simulink library "EmE_MBD_Blockset"  (R2018a)
settings: Solver=ode1  StartTime=0.0  StopTime=Inf  FixedStep=0.001  RelTol=1e-3  EnableMultiTasking=on
PostLoadFcn:
  | , if any(exist('dsrtsu_mdlpostloadfcn', 'file') == [2, 3, 6]), try dsrtsu_mdlpostloadfcn('Execute', bdroot); catch fprintf('Error in PostLoadFcn (dsrtsu_mdlpostloadfcn) for model "%s":\n %s\n', bdroot, lasterr); end, end,
undefined symbols (not defined in the file or in its folder): ENUM_TSC1_CONTROL_PURPOSE_T, gcbh, GLB_SWITCH_T
libraries: simulink x237, $bdroot x115, simulink_need_slupdate x26, MotoHawk_lib x13, simulink_extras x3
(part 11 of 11)

== system EmE_MBD_Blockset/User-Defined Functions/Snoop/CCP_ETC_SS2/CCP_Parameter_Decode/Decode_Signal7/Signal Decode/FLOAT32 ==
  note: (-1)^s × c × b^q
  note: S        Q         C
      | 31    30-23    22-0
  Raw32 : Inport
  Add8 : Sum
  Add9 : Sum  Inputs=-+
  Bitwise Operator : simulink/Logic and Bit Operations/Bitwise Operator  logicop=AND  UseBitMask=on  BitMask=bin2dec('10000000000000000000000000000000')  BitMaskRealWorld=Stored Integer
  Bitwise Operator1 : simulink/Logic and Bit Operations/Bitwise Operator  logicop=AND  UseBitMask=on  BitMask=bin2dec('01111111100000000000000000000000')  BitMaskRealWorld=Stored Integer
  Bitwise Operator2 : simulink/Logic and Bit Operations/Bitwise Operator  logicop=AND  UseBitMask=on  BitMask=bin2dec('00000000011111111111111111111111')  BitMaskRealWorld=Stored Integer
  Constant : Constant  Value=10
  Constant5 : Constant  OutDataTypeStr=double
  Constant6 : Constant  Value=2  OutDataTypeStr=double
  Constant7 : Constant  Value=127  OutDataTypeStr=double
  Data Type Conversion{1..8} (8 alike) : DataTypeConversion  OutDataTypeStr=double
  Math Function1 : Math  Operator=pow  SaturateOnIntegerOverflow=on
  Product1 : Product  RndMeth=Zero
  Shift Arithmetic6 : ArithShift
  Shift Arithmetic7 : ArithShift
  Shift Arithmetic8 : ArithShift
  Terminator3 : Terminator
  sign1 : Terminator
  Raw : Outport
  wires:
  Data Type Conversion8/1 -> Product1/1
  Data Type Conversion7/1 -> Product1/2
  Data Type Conversion6/1 -> Add8/1
  Data Type Conversion5/1 -> Add9/1
  Data Type Conversion3/1 -> Shift Arithmetic8/1
  Data Type Conversion1/1 -> Raw/1
  Product1/1 -> Data Type Conversion1/1
  Add8/1 -> Data Type Conversion7/1
  Constant7/1 -> Data Type Conversion5/1
  Data Type Conversion4/1 -> Add9/2
  Math Function1/1 -> Data Type Conversion8/1
  Constant6/1 -> Math Function1/1
  Add9/1 -> Math Function1/2
  Shift Arithmetic7/1 -> Data Type Conversion4/1
  Data Type Conversion2/1 -> Add8/2
  Constant5/1 -> Data Type Conversion6/1
  Shift Arithmetic8/1 -> Data Type Conversion2/1
  Shift Arithmetic6/1 -> sign1/1
  Bitwise Operator/1 -> Shift Arithmetic6/1  "s"
  Bitwise Operator1/1 -> Shift Arithmetic7/1  "q"
  Bitwise Operator2/1 -> Data Type Conversion3/1  "c"
  Raw32/1 -> Bitwise Operator/1, Bitwise Operator1/1, Bitwise Operator2/1
  Constant/1 -> Terminator3/1  "b"

== system EmE_MBD_Blockset/User-Defined Functions/Snoop/CCP_ETC_SS2/CCP_Parameter_Decode/Decode_Signal7/Signal Decode/Integer_Data ==
  Type : Inport
  Raw32 : Inport  Port=2
  Bitwise Operator : simulink/Logic and Bit Operations/Bitwise Operator  logicop=AND  UseBitMask=on  BitMask=bin2dec('1000')  BitMaskRealWorld=Stored Integer
  Bitwise Operator1 : simulink/Logic and Bit Operations/Bitwise Operator  logicop=AND  UseBitMask=on  BitMask=hex2dec('8000')  BitMaskRealWorld=Stored Integer
  Bitwise Operator2 : simulink/Logic and Bit Operations/Bitwise Operator  logicop=AND  UseBitMask=on  BitMask=bin2dec('0100')  BitMaskRealWorld=Stored Integer
  Bitwise Operator3 : simulink/Logic and Bit Operations/Bitwise Operator  logicop=AND  UseBitMask=on  BitMask=bin2dec('0010')  BitMaskRealWorld=Stored Integer
  Bitwise Operator5 : simulink/Logic and Bit Operations/Bitwise Operator  logicop=AND  UseBitMask=on  BitMask=hex2dec('80')  BitMaskRealWorld=Stored Integer
  Bitwise Operator6 : simulink/Logic and Bit Operations/Bitwise Operator  logicop=AND  UseBitMask=on  BitMask=hex2dec('80000000')  BitMaskRealWorld=Stored Integer
  Bitwise Operator7 : simulink/Logic and Bit Operations/Bitwise Operator  logicop=AND  UseBitMask=on  BitMask=bin2dec('0111111111111111')  BitMaskRealWorld=Stored Integer
  Bitwise Operator8 : simulink/Logic and Bit Operations/Bitwise Operator  logicop=AND  UseBitMask=on  BitMask=hex2dec('7F')  BitMaskRealWorld=Stored Integer
  Bitwise Operator9 : simulink/Logic and Bit Operations/Bitwise Operator  logicop=AND  UseBitMask=on  BitMask=hex2dec('7FFFFFF')  BitMaskRealWorld=Stored Integer
  Constant1 : Constant  Value=0  OutDataTypeStr=boolean
  Constant3 : Constant  OutDataTypeStr=boolean
  Data Type Conversion{5,9..11} (4 alike) : DataTypeConversion  OutDataTypeStr=double
  Gain : Gain  Gain=-1
  Logical Operator{,2..4} (4 alike) : Logic  AllPortsSameDT=off  OutDataTypeStr=boolean
  Logical Operator1 : Logic  Operator=NOR  AllPortsSameDT=off  OutDataTypeStr=boolean
  Logical Operator5 : Logic  Operator=OR  Inputs=3  AllPortsSameDT=off  OutDataTypeStr=boolean
  Switch{1..5} (5 alike) : Switch  Criteria=u2 ~= 0
  Raw : Outport
  wires:
  Type/1 -> Bitwise Operator/1, Bitwise Operator3/1, Bitwise Operator2/1
  Bitwise Operator/1 -> Switch1/2  "F_signed"
  Constant3/1 -> Switch1/1
  Constant1/1 -> Switch1/3
  Switch1/1 -> [f_signed]  "Sign"
  [f_signed] -> Switch4/2
  Switch5/1 -> Raw/1
  Bitwise Operator2/1 -> [F_4Byte], Logical Operator1/1  "F_4Byte"
  Bitwise Operator3/1 -> [F_2Byte], Logical Operator1/2  "F_2Byte"
  Logical Operator1/1 -> [F_1Byte]
  Bitwise Operator5/1 -> Logical Operator/2
  Bitwise Operator1/1 -> Logical Operator3/2
  Bitwise Operator6/1 -> Logical Operator4/2
  Raw32/1 -> Bitwise Operator5/1, Bitwise Operator6/1, Bitwise Operator1/1, Bitwise Operator8/1, Bitwise Operator7/1, Bitwise Operator9/1, Data Type Conversion10/1
  Bitwise Operator7/1 -> Data Type Conversion9/1
  Data Type Conversion9/1 -> Switch2/1
  [F_2Byte] -> Switch2/2
  Bitwise Operator8/1 -> Data Type Conversion5/1
  Data Type Conversion5/1 -> Switch2/3
  [F_1Byte] -> Logical Operator/1
  [F_2Byte] -> Logical Operator3/1
  [F_4Byte] -> Logical Operator4/1
  Logical Operator/1 -> Logical Operator5/1
  Logical Operator3/1 -> Logical Operator5/2
  Logical Operator4/1 -> Logical Operator5/3
  Logical Operator5/1 -> [flip_sign]  "flip_sign"
  Switch2/1 -> Switch3/3
  [F_4Byte] -> Switch3/2
  Data Type Conversion10/1 -> Switch4/3
  Bitwise Operator9/1 -> Data Type Conversion11/1
  Data Type Conversion11/1 -> Switch3/1
  Switch3/1 -> Switch4/1
  Gain/1 -> Switch5/1
  Switch4/1 -> Switch5/3, Gain/1
  Logical Operator2/1 -> Switch5/2
  [flip_sign] -> Logical Operator2/2
  [f_signed] -> Logical Operator2/1

== system EmE_MBD_Blockset/User-Defined Functions/Snoop/CCP_ETC_SS2/CCP_Parameter_Decode/Decode_Signal7/Signal Decode/Unit_Convert ==
  Raw : Inport
  Conversion : Inport  Port=2
  Add : Sum
  Divide : Product  Inputs=*/
  Product : Product  RndMeth=Zero
  Selector1 : Selector  InputPortWidth=3  IndexOptions=Index vector (dialog)  Indices=3  OutputSizes=1
  Selector2 : Selector  InputPortWidth=3  IndexOptions=Index vector (dialog)  Indices=1  OutputSizes=1
  Selector4 : Selector  InputPortWidth=3  IndexOptions=Index vector (dialog)  Indices=2  OutputSizes=1
  Scaled : Outport
  wires:
  Add/1 -> Scaled/1
  Divide/1 -> Add/1
  Product/1 -> Divide/1
  Selector2/1 -> Product/2
  Selector4/1 -> Divide/2
  Selector1/1 -> Add/2
  Conversion/1 -> Selector2/1, Selector4/1, Selector1/1
  Raw/1 -> Product/1

== system EmE_MBD_Blockset/User-Defined Functions/Snoop/CCP_ETC_SS2/CCP_Parameter_Decode/Decode_Signal8/Isolate Data/1Byte ==
  U : Inport
  Idx : Inport  Port=2
  1Byte : Selector  IndexMode=Zero-based  InputPortWidth=7  IndexOptions=Starting index (port)  Indices=1  OutputSizes=1
  Data Type Conversion : DataTypeConversion  OutDataTypeStr=uint32
  Y : Outport
  wires:
  Data Type Conversion/1 -> Y/1
  Idx/1 -> 1Byte/2
  1Byte/1 -> Data Type Conversion/1
  U/1 -> 1Byte/1

== system EmE_MBD_Blockset/User-Defined Functions/Snoop/CCP_ETC_SS2/CCP_Parameter_Decode/Decode_Signal8/Isolate Data/2Bytes ==
  U : Inport
  Idx1 : Inport  Port=2
  2Byte : Selector  IndexMode=Zero-based  InputPortWidth=7  IndexOptions=Starting index (port)  Indices=1  OutputSizes=2
  Add : Sum
  Constant : Constant  Value=5  OutDataTypeStr=uint8
  Data Type Conversion : DataTypeConversion  OutDataTypeStr=uint32
  Data Type Conversion1 : DataTypeConversion  OutDataTypeStr=uint32
  Demux : Demux  Outputs=2
  Relational Operator : RelationalOperator  Operator=<  OutDataTypeStr=boolean  RndMeth=Nearest
  Shift Arithmetic : ArithShift
  Switch1 : Switch  Criteria=u2 ~= 0
  Y : Outport
  wires:
  Switch1/1 -> 2Byte/2
  Idx1/1 -> Switch1/3, Relational Operator/2
  Relational Operator/1 -> Switch1/2
  2Byte/1 -> Data Type Conversion1/1
  Data Type Conversion1/1 -> Demux/1
  Add/1 -> Data Type Conversion/1
  Shift Arithmetic/1 -> Add/1
  Demux/1 -> Shift Arithmetic/1
  Demux/2 -> Add/2
  U/1 -> 2Byte/1
  Data Type Conversion/1 -> Y/1
  Constant/1 -> Switch1/1, Relational Operator/1

== system EmE_MBD_Blockset/User-Defined Functions/Snoop/CCP_ETC_SS2/CCP_Parameter_Decode/Decode_Signal8/Isolate Data/4Bytes ==
  U : Inport
  Idx : Inport  Port=2
  4Byte : Selector  IndexMode=Zero-based  InputPortWidth=7  IndexOptions=Starting index (port)  Indices=1  OutputSizes=4
  Add : Sum  Inputs=++++
  Constant1 : Constant  Value=3  OutDataTypeStr=uint8
  Data Type Conversion1 : DataTypeConversion  OutDataTypeStr=uint32
  Data Type Conversion2 : DataTypeConversion  OutDataTypeStr=uint32
  Demux : Demux
  Relational Operator1 : RelationalOperator  Operator=<  OutDataTypeStr=boolean  RndMeth=Nearest
  Shift Arithmetic : ArithShift
  Shift Arithmetic1 : ArithShift
  Shift Arithmetic2 : ArithShift
  Switch2 : Switch  Criteria=u2 ~= 0
  Y : Outport
  wires:
  Switch2/1 -> 4Byte/2
  Data Type Conversion2/1 -> Demux/1
  Shift Arithmetic2/1 -> Add/3
  Demux/3 -> Shift Arithmetic2/1
  Demux/4 -> Add/4
  Shift Arithmetic1/1 -> Add/2
  Add/1 -> Data Type Conversion1/1
  Shift Arithmetic/1 -> Add/1
  Demux/1 -> Shift Arithmetic/1
  Demux/2 -> Shift Arithmetic1/1
  Data Type Conversion1/1 -> Y/1
  4Byte/1 -> Data Type Conversion2/1
  U/1 -> 4Byte/1
  Idx/1 -> Switch2/3, Relational Operator1/2
  Relational Operator1/1 -> Switch2/2
  Constant1/1 -> Switch2/1, Relational Operator1/1

== system EmE_MBD_Blockset/User-Defined Functions/Snoop/CCP_ETC_SS2/CCP_Parameter_Decode/Decode_Signal8/Isolate Data/Size ==
  Type : Inport
  Bitwise Operator : simulink/Logic and Bit Operations/Bitwise Operator  logicop=AND  UseBitMask=on  BitMask=bin2dec('00000001')  BitMaskRealWorld=Stored Integer
  Bitwise Operator1 : simulink/Logic and Bit Operations/Bitwise Operator  logicop=AND  UseBitMask=on  BitMask=bin2dec('00000010')  BitMaskRealWorld=Stored Integer
  Bitwise Operator2 : simulink/Logic and Bit Operations/Bitwise Operator  logicop=AND  UseBitMask=on  BitMask=bin2dec('00000100')  BitMaskRealWorld=Stored Integer
  Constant2 : Constant  Value=2
  Constant3 : Constant
  Constant4 : Constant  Value=4
  Logical Operator : Logic  Operator=OR  AllPortsSameDT=off  OutDataTypeStr=boolean
  Logical Operator1 : Logic  Operator=NOT  AllPortsSameDT=off  OutDataTypeStr=boolean
  Switch1 : Switch  Criteria=u2 ~= 0
  Switch2 : Switch  Criteria=u2 ~= 0
  Byte_Count : Outport
  wires:
  Constant4/1 -> Switch2/1
  Switch2/1 -> Byte_Count/1
  Constant3/1 -> Switch1/3
  Constant2/1 -> Switch1/1
  Bitwise Operator1/1 -> Switch1/2
  Logical Operator1/1 -> Logical Operator/1
  Bitwise Operator2/1 -> Logical Operator/2
  Switch1/1 -> Switch2/3
  Bitwise Operator/1 -> Logical Operator1/1
  Type/1 -> Bitwise Operator/1, Bitwise Operator1/1, Bitwise Operator2/1
  Logical Operator/1 -> Switch2/2

== system EmE_MBD_Blockset/User-Defined Functions/Snoop/CCP_ETC_SS2/CCP_Parameter_Decode/Decode_Signal8/Signal Decode/FLOAT32 ==
  note: S        Q         C
      | 31    30-23    22-0
  note: (-1)^s × c × b^q
  Raw32 : Inport
  Add8 : Sum
  Add9 : Sum  Inputs=-+
  Bitwise Operator : simulink/Logic and Bit Operations/Bitwise Operator  logicop=AND  UseBitMask=on  BitMask=bin2dec('10000000000000000000000000000000')  BitMaskRealWorld=Stored Integer
  Bitwise Operator1 : simulink/Logic and Bit Operations/Bitwise Operator  logicop=AND  UseBitMask=on  BitMask=bin2dec('01111111100000000000000000000000')  BitMaskRealWorld=Stored Integer
  Bitwise Operator2 : simulink/Logic and Bit Operations/Bitwise Operator  logicop=AND  UseBitMask=on  BitMask=bin2dec('00000000011111111111111111111111')  BitMaskRealWorld=Stored Integer
  Constant : Constant  Value=10
  Constant5 : Constant  OutDataTypeStr=double
  Constant6 : Constant  Value=2  OutDataTypeStr=double
  Constant7 : Constant  Value=127  OutDataTypeStr=double
  Data Type Conversion{1..8} (8 alike) : DataTypeConversion  OutDataTypeStr=double
  Math Function1 : Math  Operator=pow  SaturateOnIntegerOverflow=on
  Product1 : Product  RndMeth=Zero
  Shift Arithmetic6 : ArithShift
  Shift Arithmetic7 : ArithShift
  Shift Arithmetic8 : ArithShift
  Terminator3 : Terminator
  sign1 : Terminator
  Raw : Outport
  wires:
  Constant/1 -> Terminator3/1  "b"
  Raw32/1 -> Bitwise Operator2/1, Bitwise Operator1/1, Bitwise Operator/1
  Bitwise Operator2/1 -> Data Type Conversion3/1  "c"
  Bitwise Operator1/1 -> Shift Arithmetic7/1  "q"
  Bitwise Operator/1 -> Shift Arithmetic6/1  "s"
  Shift Arithmetic6/1 -> sign1/1
  Shift Arithmetic8/1 -> Data Type Conversion2/1
  Constant5/1 -> Data Type Conversion6/1
  Data Type Conversion2/1 -> Add8/2
  Shift Arithmetic7/1 -> Data Type Conversion4/1
  Add9/1 -> Math Function1/2
  Constant6/1 -> Math Function1/1
  Math Function1/1 -> Data Type Conversion8/1
  Data Type Conversion4/1 -> Add9/2
  Constant7/1 -> Data Type Conversion5/1
  Add8/1 -> Data Type Conversion7/1
  Product1/1 -> Data Type Conversion1/1
  Data Type Conversion1/1 -> Raw/1
  Data Type Conversion3/1 -> Shift Arithmetic8/1
  Data Type Conversion5/1 -> Add9/1
  Data Type Conversion6/1 -> Add8/1
  Data Type Conversion7/1 -> Product1/2
  Data Type Conversion8/1 -> Product1/1

== system EmE_MBD_Blockset/User-Defined Functions/Snoop/CCP_ETC_SS2/CCP_Parameter_Decode/Decode_Signal8/Signal Decode/Integer_Data ==
  Type : Inport
  Raw32 : Inport  Port=2
  Bitwise Operator : simulink/Logic and Bit Operations/Bitwise Operator  logicop=AND  UseBitMask=on  BitMask=bin2dec('1000')  BitMaskRealWorld=Stored Integer
  Bitwise Operator1 : simulink/Logic and Bit Operations/Bitwise Operator  logicop=AND  UseBitMask=on  BitMask=hex2dec('8000')  BitMaskRealWorld=Stored Integer
  Bitwise Operator2 : simulink/Logic and Bit Operations/Bitwise Operator  logicop=AND  UseBitMask=on  BitMask=bin2dec('0100')  BitMaskRealWorld=Stored Integer
  Bitwise Operator3 : simulink/Logic and Bit Operations/Bitwise Operator  logicop=AND  UseBitMask=on  BitMask=bin2dec('0010')  BitMaskRealWorld=Stored Integer
  Bitwise Operator5 : simulink/Logic and Bit Operations/Bitwise Operator  logicop=AND  UseBitMask=on  BitMask=hex2dec('80')  BitMaskRealWorld=Stored Integer
  Bitwise Operator6 : simulink/Logic and Bit Operations/Bitwise Operator  logicop=AND  UseBitMask=on  BitMask=hex2dec('80000000')  BitMaskRealWorld=Stored Integer
  Bitwise Operator7 : simulink/Logic and Bit Operations/Bitwise Operator  logicop=AND  UseBitMask=on  BitMask=bin2dec('0111111111111111')  BitMaskRealWorld=Stored Integer
  Bitwise Operator8 : simulink/Logic and Bit Operations/Bitwise Operator  logicop=AND  UseBitMask=on  BitMask=hex2dec('7F')  BitMaskRealWorld=Stored Integer
  Bitwise Operator9 : simulink/Logic and Bit Operations/Bitwise Operator  logicop=AND  UseBitMask=on  BitMask=hex2dec('7FFFFFF')  BitMaskRealWorld=Stored Integer
  Constant1 : Constant  Value=0  OutDataTypeStr=boolean
  Constant3 : Constant  OutDataTypeStr=boolean
  Data Type Conversion{5,9..11} (4 alike) : DataTypeConversion  OutDataTypeStr=double
  Gain : Gain  Gain=-1
  Logical Operator{,2..4} (4 alike) : Logic  AllPortsSameDT=off  OutDataTypeStr=boolean
  Logical Operator1 : Logic  Operator=NOR  AllPortsSameDT=off  OutDataTypeStr=boolean
  Logical Operator5 : Logic  Operator=OR  Inputs=3  AllPortsSameDT=off  OutDataTypeStr=boolean
  Switch{1..5} (5 alike) : Switch  Criteria=u2 ~= 0
  Raw : Outport
  wires:
  [f_signed] -> Logical Operator2/1
  [flip_sign] -> Logical Operator2/2
  Logical Operator2/1 -> Switch5/2
  Switch4/1 -> Gain/1, Switch5/3
  Gain/1 -> Switch5/1
  Switch3/1 -> Switch4/1
  Data Type Conversion11/1 -> Switch3/1
  Bitwise Operator9/1 -> Data Type Conversion11/1
  Data Type Conversion10/1 -> Switch4/3
  [F_4Byte] -> Switch3/2
  Switch2/1 -> Switch3/3
  Logical Operator5/1 -> [flip_sign]  "flip_sign"
  Logical Operator4/1 -> Logical Operator5/3
  Logical Operator3/1 -> Logical Operator5/2
  Logical Operator/1 -> Logical Operator5/1
  [F_4Byte] -> Logical Operator4/1
  [F_2Byte] -> Logical Operator3/1
  [F_1Byte] -> Logical Operator/1
  Data Type Conversion5/1 -> Switch2/3
  Bitwise Operator8/1 -> Data Type Conversion5/1
  [F_2Byte] -> Switch2/2
  Data Type Conversion9/1 -> Switch2/1
  Bitwise Operator7/1 -> Data Type Conversion9/1
  Raw32/1 -> Data Type Conversion10/1, Bitwise Operator9/1, Bitwise Operator7/1, Bitwise Operator8/1, Bitwise Operator1/1, Bitwise Operator6/1, Bitwise Operator5/1
  Bitwise Operator6/1 -> Logical Operator4/2
  Bitwise Operator1/1 -> Logical Operator3/2
  Bitwise Operator5/1 -> Logical Operator/2
  Logical Operator1/1 -> [F_1Byte]
  Bitwise Operator3/1 -> Logical Operator1/2, [F_2Byte]  "F_2Byte"
  Bitwise Operator2/1 -> Logical Operator1/1, [F_4Byte]  "F_4Byte"
  Switch5/1 -> Raw/1
  [f_signed] -> Switch4/2
  Switch1/1 -> [f_signed]  "Sign"
  Constant1/1 -> Switch1/3
  Constant3/1 -> Switch1/1
  Bitwise Operator/1 -> Switch1/2  "F_signed"
  Type/1 -> Bitwise Operator2/1, Bitwise Operator3/1, Bitwise Operator/1

== system EmE_MBD_Blockset/User-Defined Functions/Snoop/CCP_ETC_SS2/CCP_Parameter_Decode/Decode_Signal8/Signal Decode/Unit_Convert ==
  Raw : Inport
  Conversion : Inport  Port=2
  Add : Sum
  Divide : Product  Inputs=*/
  Product : Product  RndMeth=Zero
  Selector1 : Selector  InputPortWidth=3  IndexOptions=Index vector (dialog)  Indices=3  OutputSizes=1
  Selector2 : Selector  InputPortWidth=3  IndexOptions=Index vector (dialog)  Indices=1  OutputSizes=1
  Selector4 : Selector  InputPortWidth=3  IndexOptions=Index vector (dialog)  Indices=2  OutputSizes=1
  Scaled : Outport
  wires:
  Raw/1 -> Product/1
  Conversion/1 -> Selector1/1, Selector4/1, Selector2/1
  Selector1/1 -> Add/2
  Selector4/1 -> Divide/2
  Selector2/1 -> Product/2
  Product/1 -> Divide/1
  Divide/1 -> Add/1
  Add/1 -> Scaled/1

== system EmE_MBD_Blockset/User-Defined Functions/Snoop/CCP_ETC_SS2/CCP_Parameter_Decode/Decode_Signal9/Isolate Data/1Byte ==
  U : Inport
  Idx : Inport  Port=2
  1Byte : Selector  IndexMode=Zero-based  InputPortWidth=7  IndexOptions=Starting index (port)  Indices=1  OutputSizes=1
  Data Type Conversion : DataTypeConversion  OutDataTypeStr=uint32
  Y : Outport
  wires:
  U/1 -> 1Byte/1
  1Byte/1 -> Data Type Conversion/1
  Idx/1 -> 1Byte/2
  Data Type Conversion/1 -> Y/1

== system EmE_MBD_Blockset/User-Defined Functions/Snoop/CCP_ETC_SS2/CCP_Parameter_Decode/Decode_Signal9/Isolate Data/2Bytes ==
  U : Inport
  Idx1 : Inport  Port=2
  2Byte : Selector  IndexMode=Zero-based  InputPortWidth=7  IndexOptions=Starting index (port)  Indices=1  OutputSizes=2
  Add : Sum
  Constant : Constant  Value=5  OutDataTypeStr=uint8
  Data Type Conversion : DataTypeConversion  OutDataTypeStr=uint32
  Data Type Conversion1 : DataTypeConversion  OutDataTypeStr=uint32
  Demux : Demux  Outputs=2
  Relational Operator : RelationalOperator  Operator=<  OutDataTypeStr=boolean  RndMeth=Nearest
  Shift Arithmetic : ArithShift
  Switch1 : Switch  Criteria=u2 ~= 0
  Y : Outport
  wires:
  Constant/1 -> Relational Operator/1, Switch1/1
  Data Type Conversion/1 -> Y/1
  U/1 -> 2Byte/1
  Demux/2 -> Add/2
  Demux/1 -> Shift Arithmetic/1
  Shift Arithmetic/1 -> Add/1
  Add/1 -> Data Type Conversion/1
  Data Type Conversion1/1 -> Demux/1
  2Byte/1 -> Data Type Conversion1/1
  Relational Operator/1 -> Switch1/2
  Idx1/1 -> Relational Operator/2, Switch1/3
  Switch1/1 -> 2Byte/2

== system EmE_MBD_Blockset/User-Defined Functions/Snoop/CCP_ETC_SS2/CCP_Parameter_Decode/Decode_Signal9/Isolate Data/4Bytes ==
  U : Inport
  Idx : Inport  Port=2
  4Byte : Selector  IndexMode=Zero-based  InputPortWidth=7  IndexOptions=Starting index (port)  Indices=1  OutputSizes=4
  Add : Sum  Inputs=++++
  Constant1 : Constant  Value=3  OutDataTypeStr=uint8
  Data Type Conversion1 : DataTypeConversion  OutDataTypeStr=uint32
  Data Type Conversion2 : DataTypeConversion  OutDataTypeStr=uint32
  Demux : Demux
  Relational Operator1 : RelationalOperator  Operator=<  OutDataTypeStr=boolean  RndMeth=Nearest
  Shift Arithmetic : ArithShift
  Shift Arithmetic1 : ArithShift
  Shift Arithmetic2 : ArithShift
  Switch2 : Switch  Criteria=u2 ~= 0
  Y : Outport
  wires:
  Constant1/1 -> Relational Operator1/1, Switch2/1
  Relational Operator1/1 -> Switch2/2
  Idx/1 -> Relational Operator1/2, Switch2/3
  U/1 -> 4Byte/1
  4Byte/1 -> Data Type Conversion2/1
  Data Type Conversion1/1 -> Y/1
  Demux/2 -> Shift Arithmetic1/1
  Demux/1 -> Shift Arithmetic/1
  Shift Arithmetic/1 -> Add/1
  Add/1 -> Data Type Conversion1/1
  Shift Arithmetic1/1 -> Add/2
  Demux/4 -> Add/4
  Demux/3 -> Shift Arithmetic2/1
  Shift Arithmetic2/1 -> Add/3
  Data Type Conversion2/1 -> Demux/1
  Switch2/1 -> 4Byte/2

== system EmE_MBD_Blockset/User-Defined Functions/Snoop/CCP_ETC_SS2/CCP_Parameter_Decode/Decode_Signal9/Isolate Data/Size ==
  Type : Inport
  Bitwise Operator : simulink/Logic and Bit Operations/Bitwise Operator  logicop=AND  UseBitMask=on  BitMask=bin2dec('00000001')  BitMaskRealWorld=Stored Integer
  Bitwise Operator1 : simulink/Logic and Bit Operations/Bitwise Operator  logicop=AND  UseBitMask=on  BitMask=bin2dec('00000010')  BitMaskRealWorld=Stored Integer
  Bitwise Operator2 : simulink/Logic and Bit Operations/Bitwise Operator  logicop=AND  UseBitMask=on  BitMask=bin2dec('00000100')  BitMaskRealWorld=Stored Integer
  Constant2 : Constant  Value=2
  Constant3 : Constant
  Constant4 : Constant  Value=4
  Logical Operator : Logic  Operator=OR  AllPortsSameDT=off  OutDataTypeStr=boolean
  Logical Operator1 : Logic  Operator=NOT  AllPortsSameDT=off  OutDataTypeStr=boolean
  Switch1 : Switch  Criteria=u2 ~= 0
  Switch2 : Switch  Criteria=u2 ~= 0
  Byte_Count : Outport
  wires:
  Logical Operator/1 -> Switch2/2
  Type/1 -> Bitwise Operator2/1, Bitwise Operator1/1, Bitwise Operator/1
  Bitwise Operator/1 -> Logical Operator1/1
  Switch1/1 -> Switch2/3
  Bitwise Operator2/1 -> Logical Operator/2
  Logical Operator1/1 -> Logical Operator/1
  Bitwise Operator1/1 -> Switch1/2
  Constant2/1 -> Switch1/1
  Constant3/1 -> Switch1/3
  Switch2/1 -> Byte_Count/1
  Constant4/1 -> Switch2/1

== system EmE_MBD_Blockset/User-Defined Functions/Snoop/CCP_ETC_SS2/CCP_Parameter_Decode/Decode_Signal9/Signal Decode/FLOAT32 ==
  note: (-1)^s × c × b^q
  note: S        Q         C
      | 31    30-23    22-0
  Raw32 : Inport
  Add8 : Sum
  Add9 : Sum  Inputs=-+
  Bitwise Operator : simulink/Logic and Bit Operations/Bitwise Operator  logicop=AND  UseBitMask=on  BitMask=bin2dec('10000000000000000000000000000000')  BitMaskRealWorld=Stored Integer
  Bitwise Operator1 : simulink/Logic and Bit Operations/Bitwise Operator  logicop=AND  UseBitMask=on  BitMask=bin2dec('01111111100000000000000000000000')  BitMaskRealWorld=Stored Integer
  Bitwise Operator2 : simulink/Logic and Bit Operations/Bitwise Operator  logicop=AND  UseBitMask=on  BitMask=bin2dec('00000000011111111111111111111111')  BitMaskRealWorld=Stored Integer
  Constant : Constant  Value=10
  Constant5 : Constant  OutDataTypeStr=double
  Constant6 : Constant  Value=2  OutDataTypeStr=double
  Constant7 : Constant  Value=127  OutDataTypeStr=double
  Data Type Conversion{1..8} (8 alike) : DataTypeConversion  OutDataTypeStr=double
  Math Function1 : Math  Operator=pow  SaturateOnIntegerOverflow=on
  Product1 : Product  RndMeth=Zero
  Shift Arithmetic6 : ArithShift
  Shift Arithmetic7 : ArithShift
  Shift Arithmetic8 : ArithShift
  Terminator3 : Terminator
  sign1 : Terminator
  Raw : Outport
  wires:
  Data Type Conversion8/1 -> Product1/1
  Data Type Conversion7/1 -> Product1/2
  Data Type Conversion6/1 -> Add8/1
  Data Type Conversion5/1 -> Add9/1
  Data Type Conversion3/1 -> Shift Arithmetic8/1
  Data Type Conversion1/1 -> Raw/1
  Product1/1 -> Data Type Conversion1/1
  Add8/1 -> Data Type Conversion7/1
  Constant7/1 -> Data Type Conversion5/1
  Data Type Conversion4/1 -> Add9/2
  Math Function1/1 -> Data Type Conversion8/1
  Constant6/1 -> Math Function1/1
  Add9/1 -> Math Function1/2
  Shift Arithmetic7/1 -> Data Type Conversion4/1
  Data Type Conversion2/1 -> Add8/2
  Constant5/1 -> Data Type Conversion6/1
  Shift Arithmetic8/1 -> Data Type Conversion2/1
  Shift Arithmetic6/1 -> sign1/1
  Bitwise Operator/1 -> Shift Arithmetic6/1  "s"
  Bitwise Operator1/1 -> Shift Arithmetic7/1  "q"
  Bitwise Operator2/1 -> Data Type Conversion3/1  "c"
  Raw32/1 -> Bitwise Operator/1, Bitwise Operator1/1, Bitwise Operator2/1
  Constant/1 -> Terminator3/1  "b"

== system EmE_MBD_Blockset/User-Defined Functions/Snoop/CCP_ETC_SS2/CCP_Parameter_Decode/Decode_Signal9/Signal Decode/Integer_Data ==
  Type : Inport
  Raw32 : Inport  Port=2
  Bitwise Operator : simulink/Logic and Bit Operations/Bitwise Operator  logicop=AND  UseBitMask=on  BitMask=bin2dec('1000')  BitMaskRealWorld=Stored Integer
  Bitwise Operator1 : simulink/Logic and Bit Operations/Bitwise Operator  logicop=AND  UseBitMask=on  BitMask=hex2dec('8000')  BitMaskRealWorld=Stored Integer
  Bitwise Operator2 : simulink/Logic and Bit Operations/Bitwise Operator  logicop=AND  UseBitMask=on  BitMask=bin2dec('0100')  BitMaskRealWorld=Stored Integer
  Bitwise Operator3 : simulink/Logic and Bit Operations/Bitwise Operator  logicop=AND  UseBitMask=on  BitMask=bin2dec('0010')  BitMaskRealWorld=Stored Integer
  Bitwise Operator5 : simulink/Logic and Bit Operations/Bitwise Operator  logicop=AND  UseBitMask=on  BitMask=hex2dec('80')  BitMaskRealWorld=Stored Integer
  Bitwise Operator6 : simulink/Logic and Bit Operations/Bitwise Operator  logicop=AND  UseBitMask=on  BitMask=hex2dec('80000000')  BitMaskRealWorld=Stored Integer
  Bitwise Operator7 : simulink/Logic and Bit Operations/Bitwise Operator  logicop=AND  UseBitMask=on  BitMask=bin2dec('0111111111111111')  BitMaskRealWorld=Stored Integer
  Bitwise Operator8 : simulink/Logic and Bit Operations/Bitwise Operator  logicop=AND  UseBitMask=on  BitMask=hex2dec('7F')  BitMaskRealWorld=Stored Integer
  Bitwise Operator9 : simulink/Logic and Bit Operations/Bitwise Operator  logicop=AND  UseBitMask=on  BitMask=hex2dec('7FFFFFF')  BitMaskRealWorld=Stored Integer
  Constant1 : Constant  Value=0  OutDataTypeStr=boolean
  Constant3 : Constant  OutDataTypeStr=boolean
  Data Type Conversion{5,9..11} (4 alike) : DataTypeConversion  OutDataTypeStr=double
  Gain : Gain  Gain=-1
  Logical Operator{,2..4} (4 alike) : Logic  AllPortsSameDT=off  OutDataTypeStr=boolean
  Logical Operator1 : Logic  Operator=NOR  AllPortsSameDT=off  OutDataTypeStr=boolean
  Logical Operator5 : Logic  Operator=OR  Inputs=3  AllPortsSameDT=off  OutDataTypeStr=boolean
  Switch{1..5} (5 alike) : Switch  Criteria=u2 ~= 0
  Raw : Outport
  wires:
  Type/1 -> Bitwise Operator/1, Bitwise Operator3/1, Bitwise Operator2/1
  Bitwise Operator/1 -> Switch1/2  "F_signed"
  Constant3/1 -> Switch1/1
  Constant1/1 -> Switch1/3
  Switch1/1 -> [f_signed]  "Sign"
  [f_signed] -> Switch4/2
  Switch5/1 -> Raw/1
  Bitwise Operator2/1 -> [F_4Byte], Logical Operator1/1  "F_4Byte"
  Bitwise Operator3/1 -> [F_2Byte], Logical Operator1/2  "F_2Byte"
  Logical Operator1/1 -> [F_1Byte]
  Bitwise Operator5/1 -> Logical Operator/2
  Bitwise Operator1/1 -> Logical Operator3/2
  Bitwise Operator6/1 -> Logical Operator4/2
  Raw32/1 -> Bitwise Operator5/1, Bitwise Operator6/1, Bitwise Operator1/1, Bitwise Operator8/1, Bitwise Operator7/1, Bitwise Operator9/1, Data Type Conversion10/1
  Bitwise Operator7/1 -> Data Type Conversion9/1
  Data Type Conversion9/1 -> Switch2/1
  [F_2Byte] -> Switch2/2
  Bitwise Operator8/1 -> Data Type Conversion5/1
  Data Type Conversion5/1 -> Switch2/3
  [F_1Byte] -> Logical Operator/1
  [F_2Byte] -> Logical Operator3/1
  [F_4Byte] -> Logical Operator4/1
  Logical Operator/1 -> Logical Operator5/1
  Logical Operator3/1 -> Logical Operator5/2
  Logical Operator4/1 -> Logical Operator5/3
  Logical Operator5/1 -> [flip_sign]  "flip_sign"
  Switch2/1 -> Switch3/3
  [F_4Byte] -> Switch3/2
  Data Type Conversion10/1 -> Switch4/3
  Bitwise Operator9/1 -> Data Type Conversion11/1
  Data Type Conversion11/1 -> Switch3/1
  Switch3/1 -> Switch4/1
  Gain/1 -> Switch5/1
  Switch4/1 -> Switch5/3, Gain/1
  Logical Operator2/1 -> Switch5/2
  [flip_sign] -> Logical Operator2/2
  [f_signed] -> Logical Operator2/1

== system EmE_MBD_Blockset/User-Defined Functions/Snoop/CCP_ETC_SS2/CCP_Parameter_Decode/Decode_Signal9/Signal Decode/Unit_Convert ==
  Raw : Inport
  Conversion : Inport  Port=2
  Add : Sum
  Divide : Product  Inputs=*/
  Product : Product  RndMeth=Zero
  Selector1 : Selector  InputPortWidth=3  IndexOptions=Index vector (dialog)  Indices=3  OutputSizes=1
  Selector2 : Selector  InputPortWidth=3  IndexOptions=Index vector (dialog)  Indices=1  OutputSizes=1
  Selector4 : Selector  InputPortWidth=3  IndexOptions=Index vector (dialog)  Indices=2  OutputSizes=1
  Scaled : Outport
  wires:
  Add/1 -> Scaled/1
  Divide/1 -> Add/1
  Product/1 -> Divide/1
  Selector2/1 -> Product/2
  Selector4/1 -> Divide/2
  Selector1/1 -> Add/2
  Conversion/1 -> Selector2/1, Selector4/1, Selector1/1
  Raw/1 -> Product/1

== stateflow chart EmE_MBD_Blockset/Discontinuities/Debounce/Debounce_state_machine ==
  settings: enableNonTerminalStates=1
  state WAIT
    state TO_ON
    state TO_OFF
  state OFF
    en:
    F_Out = false;
  state ON
    en:
    F_Out = true
  (default) -> OFF
  OFF -> TO_ON : [F_In]
  TO_ON -> ON [order 2] : [F_On_timer_complete]
  TO_ON -> OFF [order 1] : [~F_In]
  TO_OFF -> OFF [order 2] : [F_Off_timer_complete]
  ON -> TO_OFF : [~F_In]
  TO_OFF -> ON [order 1] : [F_In]
  data: F_In input; F_On_timer_complete input; F_Off_timer_complete input; F_Out output double
